simulink model "Lab_6_QRD_MVMUL"  (R2021a)
settings: Solver=VariableStepAuto  StartTime=0.0  StopTime=double(sim_length)  RelTol=1e-3
undefined symbols (not defined in the file or in its folder): AXI4, Lite
libraries: hdlBasic x118, xbsIndex_r4 x1
settings Model: Creator=ckk5  LastModifiedBy=ckk5

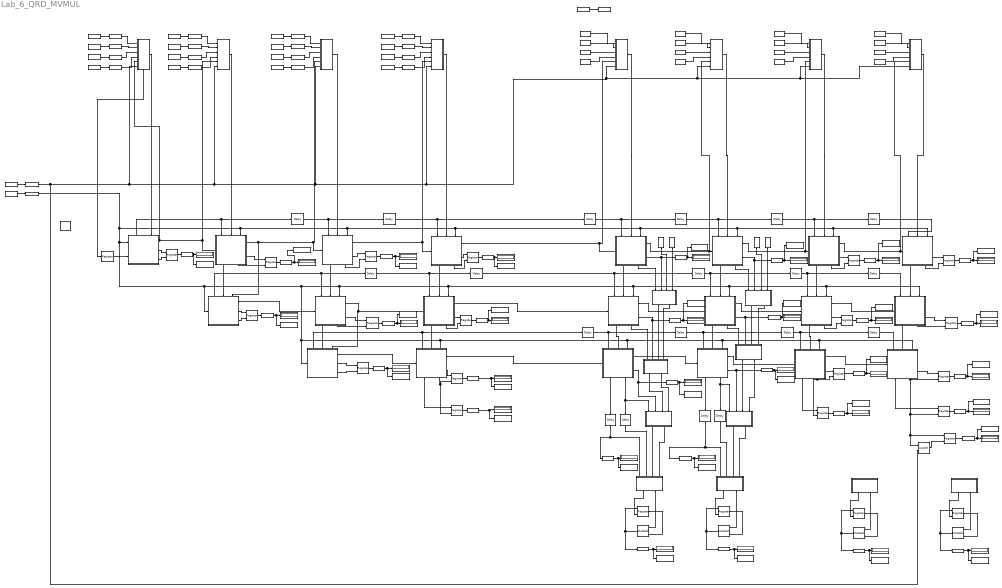
== system Lab_6_QRD_MVMUL ==
  " System Generator" : xbsIndex_r4/ System Generator  Tag=genX  xilinxfamily=zynq  part=xc7z020  speed=-1  package=clg484  synthesis_tool=Vivado  clock_wrapper=Clock Enables  directory=./netlist  proj_type=Vivado  Synth_file=Vivado Synthesis Defaults  Impl_file=Vivado Implementation Defaults  testbench=off  simulink_period=1  sysclk_period=10  dcm_input_clock_period=10  incr_netlist=off  trim_vbits=Everywhere in SubSystem  dbl_ovrd=According to Block Masks  core_generation=According to Block Masks  run_coregen=off  deprecated_control=off  eval_field=0  block_type=sysgen
  B_1 : hdlBasic/Gateway In  gui_display_data_type=Fixed-point  arith_type=Signed (2's comp)  n_bits=16  bin_pt=12  preci_type=Single  exp_width=8  frac_width=24  rows=1  columns=1  quantization="Round  (unbiased: +/- Inf)"  overflow=Saturate  period=1  UseAsADC=off  ADCChannel='1'  interface=AXI4-Lite  automatic_assignment=on  address_offset=hex2dec('00')  intf_name='array_input'  intf_description=''  default_value=0  timing_constraint=None  locs_specified=off  LOCs={}  io_standard={}  inherit_from_input=off  hdl_port=on  XmcBlockStatus=1  maskContainerNames=group4  block_type=gatewayin  block_config=sysgen:gateway_in_config  block_width_w=590  block_height_w=620  block_width=640  block_height=850
  C_{1..4} (4 alike) : hdlBasic/Gateway Out  inherit_from_input=off  hdl_port=off  rows=1  columns=1  UseAsDAC=off  DACChannel='1'  interface=AXI4-Lite  automatic_assignment=on  address_offset=hex2dec('00')  intf_name='output'  intf_description=''  timing_constraint=None  locs_specified=off  LOCs={}  io_standard={}  XmcBlockStatus=1  maskContainerNames=group4  block_type=gatewayout  block_config=sysgen:gateway_out_config  block_width_w=590  block_height_w=620  block_width=620  block_height=750
  Constant : hdlBasic/Constant  const=1.0  gui_display_data_type=Fixed-point  arith_type=Signed (2's comp)  n_bits=16  bin_pt=12  preci_type=Single  exp_width=8  frac_width=24  explicit_period=off  period=1  XmcBlockStatus=1  maskContainerNames=tabcontainer1  block_type=constant  block_config=sysgen:Constant_config
  Constant{1..4,6..9,11..14,17,19} (14 alike) : hdlBasic/Constant  const=0  gui_display_data_type=Fixed-point  arith_type=Signed (2's comp)  n_bits=16  bin_pt=12  preci_type=Single  exp_width=8  frac_width=24  explicit_period=off  period=1  XmcBlockStatus=1  maskContainerNames=tabcontainer1  block_type=constant  block_config=sysgen:Constant_config
  Constant10 : hdlBasic/Constant  const=1  gui_display_data_type=Fixed-point  arith_type=Signed (2's comp)  n_bits=16  bin_pt=12  preci_type=Single  exp_width=8  frac_width=24  explicit_period=off  period=1  XmcBlockStatus=1  maskContainerNames=tabcontainer1  block_type=constant  block_config=sysgen:Constant_config
  Constant15 : hdlBasic/Constant  const=1  gui_display_data_type=Fixed-point  arith_type=Signed (2's comp)  n_bits=16  bin_pt=12  preci_type=Single  exp_width=8  frac_width=24  explicit_period=off  period=1  XmcBlockStatus=1  maskContainerNames=tabcontainer1  block_type=constant  block_config=sysgen:Constant_config
  Constant16 : hdlBasic/Constant  const=0  gui_display_data_type=Boolean  arith_type=Boolean  n_bits=16  bin_pt=12  preci_type=Single  exp_width=8  frac_width=24  explicit_period=off  period=1  XmcBlockStatus=1  maskContainerNames=tabcontainer1  block_type=constant  block_config=sysgen:Constant_config
  Constant18 : hdlBasic/Constant  const=0  gui_display_data_type=Boolean  arith_type=Boolean  n_bits=16  bin_pt=12  preci_type=Single  exp_width=8  frac_width=24  explicit_period=off  period=1  XmcBlockStatus=1  maskContainerNames=tabcontainer1  block_type=constant  block_config=sysgen:Constant_config
  Constant5 : hdlBasic/Constant  const=1  gui_display_data_type=Fixed-point  arith_type=Signed (2's comp)  n_bits=16  bin_pt=12  preci_type=Single  exp_width=8  frac_width=24  explicit_period=off  period=1  XmcBlockStatus=1  maskContainerNames=tabcontainer1  block_type=constant  block_config=sysgen:Constant_config
  Delay{,1,4,14} (4 alike) : hdlBasic/Delay  rst=off  en=off  latency=1  reg_retiming=off  XmcBlockStatus=1  maskContainerNames=group1  block_type=delay  block_config=sysgen:Delay_config
  Delay{2..3,5..13,18..21} (15 alike) : hdlBasic/Delay  rst=off  en=off  latency=unit_L  reg_retiming=off  XmcBlockStatus=1  maskContainerNames=group1  block_type=delay  block_config=sysgen:Delay_config
  Display{,1..30} (31 alike) : Display
  From Workspace : FromWorkspace  VariableName=ap_rst  OutputAfterFinalValue=Setting to zero
  From Workspace1 : FromWorkspace  VariableName=start_new  OutputAfterFinalValue=Setting to zero
  From Workspace10 : FromWorkspace  VariableName=in_41  OutputAfterFinalValue=Setting to zero
  From Workspace11 : FromWorkspace  VariableName=in_22  OutputAfterFinalValue=Setting to zero
  From Workspace12 : FromWorkspace  VariableName=in_32  OutputAfterFinalValue=Setting to zero
  From Workspace13 : FromWorkspace  VariableName=in_33  OutputAfterFinalValue=Setting to zero
  From Workspace14 : FromWorkspace  VariableName=in_44  OutputAfterFinalValue=Setting to zero
  From Workspace15 : FromWorkspace  VariableName=in_14  OutputAfterFinalValue=Setting to zero
  From Workspace16 : FromWorkspace  VariableName=in_24  OutputAfterFinalValue=Setting to zero
  From Workspace17 : FromWorkspace  VariableName=in_34  OutputAfterFinalValue=Setting to zero
  From Workspace18 : FromWorkspace  VariableName=B_1  OutputAfterFinalValue=Setting to zero
  From Workspace2 : FromWorkspace  VariableName=in_43  OutputAfterFinalValue=Setting to zero
  From Workspace3 : FromWorkspace  VariableName=in_42  OutputAfterFinalValue=Setting to zero
  From Workspace4 : FromWorkspace  VariableName=in_13  OutputAfterFinalValue=Setting to zero
  From Workspace5 : FromWorkspace  VariableName=in_23  OutputAfterFinalValue=Setting to zero
  From Workspace6 : FromWorkspace  VariableName=in_11  OutputAfterFinalValue=Setting to zero
  From Workspace7 : FromWorkspace  VariableName=in_12  OutputAfterFinalValue=Setting to zero
  From Workspace8 : FromWorkspace  VariableName=in_21  OutputAfterFinalValue=Setting to zero
  From Workspace9 : FromWorkspace  VariableName=in_31  OutputAfterFinalValue=Setting to zero
  Logical3 : hdlBasic/Logical  logical_function=OR  inputs=2  en=off  latency=0  precision=Full  arith_type=Unsigned  n_bits=16  bin_pt=0  align_bp=on  overflow=[]  quantization=[]  XmcBlockStatus=1  maskContainerNames=tabcontainer1  block_type=logical  block_config=sysgen:Logical_config
  MultAdd{,1..3} (4 alike) : hdlBasic/MultAdd  mode=Addition  en=off  latency=0  precision=Full  arith_type=Unsigned  n_bits=16  bin_pt=14  XmcBlockStatus=1  maskContainerNames=tabcontainer1  block_type=multadd  block_config=sysgen:MultAdd_config
  Q_1 : hdlBasic/Gateway Out  inherit_from_input=off  hdl_port=on  rows=1  columns=1  UseAsDAC=off  DACChannel='1'  interface=AXI4-Lite  automatic_assignment=on  address_offset=hex2dec('00')  intf_name='control'  intf_description=''  timing_constraint=None  locs_specified=off  LOCs={}  io_standard={}  XmcBlockStatus=1  maskContainerNames=group4  block_type=gatewayout  block_config=sysgen:gateway_out_config  block_width_w=590  block_height_w=620  block_width=620  block_height=750
  Q_{11,21..22,31..32,41} (6 alike) : hdlBasic/Gateway Out  inherit_from_input=off  hdl_port=off  rows=1  columns=1  UseAsDAC=off  DACChannel='1'  interface=None  automatic_assignment=on  address_offset=hex2dec('00')  intf_name='output'  intf_description=''  timing_constraint=None  locs_specified=off  LOCs={}  io_standard={}  XmcBlockStatus=1  maskContainerNames=group4  block_type=gatewayout  block_config=sysgen:gateway_out_config  block_width_w=590  block_height_w=620  block_width=620  block_height=750
  Q_{12..14,23..24,33..34,43..44} (9 alike) : hdlBasic/Gateway Out  inherit_from_input=off  hdl_port=on  rows=1  columns=1  UseAsDAC=off  DACChannel='1'  interface=AXI4-Lite  automatic_assignment=on  address_offset=hex2dec('00')  intf_name='output'  intf_description=''  timing_constraint=None  locs_specified=off  LOCs={}  io_standard={}  XmcBlockStatus=1  maskContainerNames=group4  block_type=gatewayout  block_config=sysgen:gateway_out_config  block_width_w=590  block_height_w=620  block_width=620  block_height=750
  Q_42 : hdlBasic/Gateway Out  inherit_from_input=off  hdl_port=off  rows=1  columns=1  UseAsDAC=off  DACChannel='1'  interface=None  automatic_assignment=off  address_offset=hex2dec('00')  intf_name='output'  intf_description=''  timing_constraint=None  locs_specified=off  LOCs={}  io_standard={}  XmcBlockStatus=1  maskContainerNames=group4  block_type=gatewayout  block_config=sysgen:gateway_out_config  block_width_w=590  block_height_w=620  block_width=620  block_height=750
  R_{11..14,22..24,33..34,44} (10 alike) : hdlBasic/Gateway Out  inherit_from_input=off  hdl_port=on  rows=1  columns=1  UseAsDAC=off  DACChannel='1'  interface=AXI4-Lite  automatic_assignment=on  address_offset=hex2dec('00')  intf_name='output'  intf_description=''  timing_constraint=None  locs_specified=off  LOCs={}  io_standard={}  XmcBlockStatus=1  maskContainerNames=group4  block_type=gatewayout  block_config=sysgen:gateway_out_config  block_width_w=590  block_height_w=620  block_width=620  block_height=750
  Register{,1..4,6..14,16..18,20..21,24..25,27..28} (23 alike) : hdlBasic/Register  init=0  rst=off  en=on  XmcBlockStatus=1  maskContainerNames=tabcontainer1  block_type=register  block_config=sysgen:Register_config
  Register26 : hdlBasic/Register  init=0  rst=off  en=off  XmcBlockStatus=1  maskContainerNames=tabcontainer1  block_type=register  block_config=sysgen:Register_config
  Subsystem{,1..7} (8 alike) : Subsystem  ReferencedSubsystem=input_muxer
      Subsystem settings: PortSchema="{\"entries\":[{\"content\":{\"sides\":[{\"content\":{\"connectorIds\":[\"In1\",\"In2\",\"In3\",\"In4\",\"In5\",\"In6\"]},\"type\":\"ConnectorPlacement.EquallySpacedRectSide\",\"uuid\":\"c9659870-197e-4708-9e56-aa8d60ec2132\"},{\"content\":{\"connectorIds\":[\"Out1\"],\"side\":\"RIGHT\"},\"type\":\"ConnectorPlacement.EquallySpacedRectSide\",\"uuid\":\"f9d7c189-098f-4a24-828d-c7ef82e0ce16\"},{\"content\":{\"connectorIds\":[],\"side\":\"TOP\"},\"type\":\"ConnectorPlacement.EquallySpacedRectSide\",\"uuid\":\"5053940a-c387-4687-a81e-c4b094664b8d\"},{\"content\":{\"connectorIds\":[\"Out2\"],\"side\":\"BOTTOM\"},\"type\":\"ConnectorPlacement.EquallySpacedRectSide\",\"uuid\":\"4f75bbb3-aea6-4cac-bddf-f1fd262beda3\"}]},\"type\":\"ConnectorPlacement.EquallySpacedConnector\",\"uuid\":\"5b5beda6-ba80-4093-9766-00cb89766bfd\"}],\"packageUris\":[\"http://schema.mathworks.com/mf0/Connector/R2020b\"],\"version\":\"1.0\"}"
      Subsystem1 settings: PortSchema="{\"entries\":[{\"content\":{\"sides\":[{\"content\":{\"connectorIds\":[\"In1\",\"In2\",\"In3\",\"In4\",\"In5\",\"In6\"]},\"type\":\"ConnectorPlacement.EquallySpacedRectSide\",\"uuid\":\"c9659870-197e-4708-9e56-aa8d60ec2132\"},{\"content\":{\"connectorIds\":[\"Out1\"],\"side\":\"RIGHT\"},\"type\":\"ConnectorPlacement.EquallySpacedRectSide\",\"uuid\":\"f9d7c189-098f-4a24-828d-c7ef82e0ce16\"},{\"content\":{\"connectorIds\":[],\"side\":\"TOP\"},\"type\":\"ConnectorPlacement.EquallySpacedRectSide\",\"uuid\":\"5053940a-c387-4687-a81e-c4b094664b8d\"},{\"content\":{\"connectorIds\":[\"Out2\"],\"side\":\"BOTTOM\"},\"type\":\"ConnectorPlacement.EquallySpacedRectSide\",\"uuid\":\"0386b525-0d84-489d-b1ba-c0f65ef89545\"}]},\"type\":\"ConnectorPlacement.EquallySpacedConnector\",\"uuid\":\"5b5beda6-ba80-4093-9766-00cb89766bfd\"}],\"packageUris\":[\"http://schema.mathworks.com/mf0/Connector/R2020b\"],\"version\":\"1.0\"}"
      Subsystem2 settings: PortSchema="{\"entries\":[{\"content\":{\"sides\":[{\"content\":{\"connectorIds\":[\"In1\",\"In2\",\"In3\",\"In4\",\"In5\",\"In6\"]},\"type\":\"ConnectorPlacement.EquallySpacedRectSide\",\"uuid\":\"c9659870-197e-4708-9e56-aa8d60ec2132\"},{\"content\":{\"connectorIds\":[\"Out1\"],\"side\":\"RIGHT\"},\"type\":\"ConnectorPlacement.EquallySpacedRectSide\",\"uuid\":\"f9d7c189-098f-4a24-828d-c7ef82e0ce16\"},{\"content\":{\"connectorIds\":[],\"side\":\"TOP\"},\"type\":\"ConnectorPlacement.EquallySpacedRectSide\",\"uuid\":\"5053940a-c387-4687-a81e-c4b094664b8d\"},{\"content\":{\"connectorIds\":[\"Out2\"],\"side\":\"BOTTOM\"},\"type\":\"ConnectorPlacement.EquallySpacedRectSide\",\"uuid\":\"0b7a346d-dc43-4519-a9aa-7889b337343a\"}]},\"type\":\"ConnectorPlacement.EquallySpacedConnector\",\"uuid\":\"5b5beda6-ba80-4093-9766-00cb89766bfd\"}],\"packageUris\":[\"http://schema.mathworks.com/mf0/Connector/R2020b\"],\"version\":\"1.0\"}"
      Subsystem3 settings: PortSchema="{\"entries\":[{\"content\":{\"sides\":[{\"content\":{\"connectorIds\":[\"In1\",\"In2\",\"In3\",\"In4\",\"In5\",\"In6\"]},\"type\":\"ConnectorPlacement.EquallySpacedRectSide\",\"uuid\":\"c9659870-197e-4708-9e56-aa8d60ec2132\"},{\"content\":{\"connectorIds\":[\"Out1\"],\"side\":\"RIGHT\"},\"type\":\"ConnectorPlacement.EquallySpacedRectSide\",\"uuid\":\"f9d7c189-098f-4a24-828d-c7ef82e0ce16\"},{\"content\":{\"connectorIds\":[],\"side\":\"TOP\"},\"type\":\"ConnectorPlacement.EquallySpacedRectSide\",\"uuid\":\"5053940a-c387-4687-a81e-c4b094664b8d\"},{\"content\":{\"connectorIds\":[\"Out2\"],\"side\":\"BOTTOM\"},\"type\":\"ConnectorPlacement.EquallySpacedRectSide\",\"uuid\":\"96ca4152-851a-4b7b-aabe-a144e8b0fd46\"}]},\"type\":\"ConnectorPlacement.EquallySpacedConnector\",\"uuid\":\"5b5beda6-ba80-4093-9766-00cb89766bfd\"}],\"packageUris\":[\"http://schema.mathworks.com/mf0/Connector/R2020b\"],\"version\":\"1.0\"}"
      Subsystem4 settings: PortSchema="{\"entries\":[{\"content\":{\"sides\":[{\"content\":{\"connectorIds\":[\"In1\",\"In2\",\"In3\",\"In4\",\"In5\",\"In6\"]},\"type\":\"ConnectorPlacement.EquallySpacedRectSide\",\"uuid\":\"c9659870-197e-4708-9e56-aa8d60ec2132\"},{\"content\":{\"connectorIds\":[\"Out1\"],\"side\":\"RIGHT\"},\"type\":\"ConnectorPlacement.EquallySpacedRectSide\",\"uuid\":\"f9d7c189-098f-4a24-828d-c7ef82e0ce16\"},{\"content\":{\"connectorIds\":[],\"side\":\"TOP\"},\"type\":\"ConnectorPlacement.EquallySpacedRectSide\",\"uuid\":\"5053940a-c387-4687-a81e-c4b094664b8d\"},{\"content\":{\"connectorIds\":[\"Out2\"],\"side\":\"BOTTOM\"},\"type\":\"ConnectorPlacement.EquallySpacedRectSide\",\"uuid\":\"96ca4152-851a-4b7b-aabe-a144e8b0fd46\"}]},\"type\":\"ConnectorPlacement.EquallySpacedConnector\",\"uuid\":\"5b5beda6-ba80-4093-9766-00cb89766bfd\"}],\"packageUris\":[\"http://schema.mathworks.com/mf0/Connector/R2020b\"],\"version\":\"1.0\"}"
      Subsystem5 settings: PortSchema="{\"entries\":[{\"content\":{\"sides\":[{\"content\":{\"connectorIds\":[\"In1\",\"In2\",\"In3\",\"In4\",\"In5\",\"In6\"]},\"type\":\"ConnectorPlacement.EquallySpacedRectSide\",\"uuid\":\"c9659870-197e-4708-9e56-aa8d60ec2132\"},{\"content\":{\"connectorIds\":[\"Out1\"],\"side\":\"RIGHT\"},\"type\":\"ConnectorPlacement.EquallySpacedRectSide\",\"uuid\":\"f9d7c189-098f-4a24-828d-c7ef82e0ce16\"},{\"content\":{\"connectorIds\":[],\"side\":\"TOP\"},\"type\":\"ConnectorPlacement.EquallySpacedRectSide\",\"uuid\":\"5053940a-c387-4687-a81e-c4b094664b8d\"},{\"content\":{\"connectorIds\":[\"Out2\"],\"side\":\"BOTTOM\"},\"type\":\"ConnectorPlacement.EquallySpacedRectSide\",\"uuid\":\"96ca4152-851a-4b7b-aabe-a144e8b0fd46\"}]},\"type\":\"ConnectorPlacement.EquallySpacedConnector\",\"uuid\":\"5b5beda6-ba80-4093-9766-00cb89766bfd\"}],\"packageUris\":[\"http://schema.mathworks.com/mf0/Connector/R2020b\"],\"version\":\"1.0\"}"
      Subsystem6 settings: PortSchema="{\"entries\":[{\"content\":{\"sides\":[{\"content\":{\"connectorIds\":[\"In1\",\"In2\",\"In3\",\"In4\",\"In5\",\"In6\"]},\"type\":\"ConnectorPlacement.EquallySpacedRectSide\",\"uuid\":\"c9659870-197e-4708-9e56-aa8d60ec2132\"},{\"content\":{\"connectorIds\":[\"Out1\"],\"side\":\"RIGHT\"},\"type\":\"ConnectorPlacement.EquallySpacedRectSide\",\"uuid\":\"f9d7c189-098f-4a24-828d-c7ef82e0ce16\"},{\"content\":{\"connectorIds\":[],\"side\":\"TOP\"},\"type\":\"ConnectorPlacement.EquallySpacedRectSide\",\"uuid\":\"5053940a-c387-4687-a81e-c4b094664b8d\"},{\"content\":{\"connectorIds\":[\"Out2\"],\"side\":\"BOTTOM\"},\"type\":\"ConnectorPlacement.EquallySpacedRectSide\",\"uuid\":\"96ca4152-851a-4b7b-aabe-a144e8b0fd46\"}]},\"type\":\"ConnectorPlacement.EquallySpacedConnector\",\"uuid\":\"5b5beda6-ba80-4093-9766-00cb89766bfd\"}],\"packageUris\":[\"http://schema.mathworks.com/mf0/Connector/R2020b\"],\"version\":\"1.0\"}"
      Subsystem7 settings: PortSchema="{\"entries\":[{\"content\":{\"sides\":[{\"content\":{\"connectorIds\":[\"In1\",\"In2\",\"In3\",\"In4\",\"In5\",\"In6\"]},\"type\":\"ConnectorPlacement.EquallySpacedRectSide\",\"uuid\":\"c9659870-197e-4708-9e56-aa8d60ec2132\"},{\"content\":{\"connectorIds\":[\"Out1\"],\"side\":\"RIGHT\"},\"type\":\"ConnectorPlacement.EquallySpacedRectSide\",\"uuid\":\"f9d7c189-098f-4a24-828d-c7ef82e0ce16\"},{\"content\":{\"connectorIds\":[],\"side\":\"TOP\"},\"type\":\"ConnectorPlacement.EquallySpacedRectSide\",\"uuid\":\"5053940a-c387-4687-a81e-c4b094664b8d\"},{\"content\":{\"connectorIds\":[\"Out2\"],\"side\":\"BOTTOM\"},\"type\":\"ConnectorPlacement.EquallySpacedRectSide\",\"uuid\":\"96ca4152-851a-4b7b-aabe-a144e8b0fd46\"}]},\"type\":\"ConnectorPlacement.EquallySpacedConnector\",\"uuid\":\"5b5beda6-ba80-4093-9766-00cb89766bfd\"}],\"packageUris\":[\"http://schema.mathworks.com/mf0/Connector/R2020b\"],\"version\":\"1.0\"}"
  Subsystem Reference : Subsystem  ReferencedSubsystem=ATAN_static
      settings: PortSchema="{\"entries\":[{\"content\":{\"sides\":[{\"content\":{\"connectorIds\":[\"In1\"]},\"type\":\"ConnectorPlacement.EquallySpacedRectSide\",\"uuid\":\"e73d0d7d-03bc-4d00-801b-b8c760b16be4\"},{\"content\":{\"connectorIds\":[\"Out1\",\"Out3\",\"Out4\"],\"side\":\"RIGHT\"},\"type\":\"ConnectorPlacement.EquallySpacedRectSide\",\"uuid\":\"fb412951-8b1f-47f8-8fed-40e91e78b205\"},{\"content\":{\"connectorIds\":[\"Out2\",\"In3\",\"In2\"],\"side\":\"TOP\"},\"type\":\"ConnectorPlacement.EquallySpacedRectSide\",\"uuid\":\"8225374e-1161-490d-99ec-3bdc7c7ef343\"},{\"content\":{\"connectorIds\":[\"Out5\"],\"side\":\"BOTTOM\"},\"type\":\"ConnectorPlacement.EquallySpacedRectSide\",\"uuid\":\"cef28eec-a681-4ab7-b320-ffc64443d109\"}]},\"type\":\"ConnectorPlacement.EquallySpacedConnector\",\"uuid\":\"16b5b7a4-aca7-4d8e-a872-8aaff24fa59b\"}],\"packageUris\":[\"http://schema.mathworks.com/mf0/Connector/R2020b\"],\"version\":\"1.0\"}"
  Subsystem Reference1 : Subsystem  ReferencedSubsystem=ATAN_static
      settings: PortSchema="{\"entries\":[{\"content\":{\"sides\":[{\"content\":{\"connectorIds\":[\"In1\",\"In2\"]},\"type\":\"ConnectorPlacement.EquallySpacedRectSide\",\"uuid\":\"e73d0d7d-03bc-4d00-801b-b8c760b16be4\"},{\"content\":{\"connectorIds\":[\"Out1\",\"Out3\",\"Out4\"],\"side\":\"RIGHT\"},\"type\":\"ConnectorPlacement.EquallySpacedRectSide\",\"uuid\":\"fb412951-8b1f-47f8-8fed-40e91e78b205\"},{\"content\":{\"connectorIds\":[\"Out2\",\"In3\"],\"side\":\"TOP\"},\"type\":\"ConnectorPlacement.EquallySpacedRectSide\",\"uuid\":\"8225374e-1161-490d-99ec-3bdc7c7ef343\"},{\"content\":{\"connectorIds\":[\"Out5\"],\"side\":\"BOTTOM\"},\"type\":\"ConnectorPlacement.EquallySpacedRectSide\",\"uuid\":\"cef28eec-a681-4ab7-b320-ffc64443d109\"}]},\"type\":\"ConnectorPlacement.EquallySpacedConnector\",\"uuid\":\"16b5b7a4-aca7-4d8e-a872-8aaff24fa59b\"}],\"packageUris\":[\"http://schema.mathworks.com/mf0/Connector/R2020b\"],\"version\":\"1.0\"}"
  Subsystem Reference{2,4..20} (18 alike) : Subsystem  ReferencedSubsystem=ROT_static
      settings: PortSchema="{\"entries\":[{\"content\":{\"sides\":[{\"content\":{\"connectorIds\":[\"In2\"]},\"type\":\"ConnectorPlacement.EquallySpacedRectSide\",\"uuid\":\"e73d0d7d-03bc-4d00-801b-b8c760b16be4\"},{\"content\":{\"connectorIds\":[\"Out1\",\"Out3\"],\"side\":\"RIGHT\"},\"type\":\"ConnectorPlacement.EquallySpacedRectSide\",\"uuid\":\"fb412951-8b1f-47f8-8fed-40e91e78b205\"},{\"content\":{\"connectorIds\":[\"In3\",\"In4\",\"In1\"],\"side\":\"TOP\"},\"type\":\"ConnectorPlacement.EquallySpacedRectSide\",\"uuid\":\"8225374e-1161-490d-99ec-3bdc7c7ef343\"},{\"content\":{\"connectorIds\":[\"Out2\",\"Out4\"],\"side\":\"BOTTOM\"},\"type\":\"ConnectorPlacement.EquallySpacedRectSide\",\"uuid\":\"cef28eec-a681-4ab7-b320-ffc64443d109\"}]},\"type\":\"ConnectorPlacement.EquallySpacedConnector\",\"uuid\":\"16b5b7a4-aca7-4d8e-a872-8aaff24fa59b\"}],\"packageUris\":[\"http://schema.mathworks.com/mf0/Connector/R2020b\"],\"version\":\"1.0\"}"
  Subsystem Reference3 : Subsystem  ReferencedSubsystem=ATAN_static
      settings: PortSchema="{\"entries\":[{\"content\":{\"sides\":[{\"content\":{\"connectorIds\":[\"In1\"]},\"type\":\"ConnectorPlacement.EquallySpacedRectSide\",\"uuid\":\"e73d0d7d-03bc-4d00-801b-b8c760b16be4\"},{\"content\":{\"connectorIds\":[\"Out1\",\"Out3\",\"Out4\"],\"side\":\"RIGHT\"},\"type\":\"ConnectorPlacement.EquallySpacedRectSide\",\"uuid\":\"fb412951-8b1f-47f8-8fed-40e91e78b205\"},{\"content\":{\"connectorIds\":[\"Out2\",\"In3\",\"In2\"],\"side\":\"TOP\"},\"type\":\"ConnectorPlacement.EquallySpacedRectSide\",\"uuid\":\"8225374e-1161-490d-99ec-3bdc7c7ef343\"},{\"content\":{\"connectorIds\":[\"Out5\"],\"side\":\"BOTTOM\"},\"type\":\"ConnectorPlacement.EquallySpacedRectSide\",\"uuid\":\"cef28eec-a681-4ab7-b320-ffc64443d109\"}]},\"type\":\"ConnectorPlacement.EquallySpacedConnector\",\"uuid\":\"16b5b7a4-aca7-4d8e-a872-8aaff24fa59b\"}],\"packageUris\":[\"http://schema.mathworks.com/mf0/Connector/R2020b\"],\"version\":\"1.0\"}"
  Subsystem{8..17} (10 alike) : Subsystem  ReferencedSubsystem=Output_Selector_Simple
      Subsystem10 settings: PortSchema="{\"entries\":[{\"content\":{\"sides\":[{\"content\":{\"connectorIds\":[]},\"type\":\"ConnectorPlacement.EquallySpacedRectSide\",\"uuid\":\"f96c7e86-64a4-4252-abea-b711e367158a\"},{\"content\":{\"connectorIds\":[],\"side\":\"RIGHT\"},\"type\":\"ConnectorPlacement.EquallySpacedRectSide\",\"uuid\":\"0939b534-8e75-43bd-89b2-3b8c6cf8d932\"},{\"content\":{\"connectorIds\":[\"In2\",\"In1\",\"In4\",\"In3\"],\"side\":\"TOP\"},\"type\":\"ConnectorPlacement.EquallySpacedRectSide\",\"uuid\":\"1f2daeb6-2bdf-409b-a45b-4c9e00127dcc\"},{\"content\":{\"connectorIds\":[\"Out2\",\"Out1\"],\"side\":\"BOTTOM\"},\"type\":\"ConnectorPlacement.EquallySpacedRectSide\",\"uuid\":\"39a7ca2e-4955-4af4-a4e8-230b89e841c3\"}]},\"type\":\"ConnectorPlacement.EquallySpacedConnector\",\"uuid\":\"4fbf931e-4755-4fcf-8161-08b087bf3058\"}],\"packageUris\":[\"http://schema.mathworks.com/mf0/Connector/R2020b\"],\"version\":\"1.0\"}"
      Subsystem11 settings: PortSchema="{\"entries\":[{\"content\":{\"sides\":[{\"content\":{\"connectorIds\":[]},\"type\":\"ConnectorPlacement.EquallySpacedRectSide\",\"uuid\":\"f96c7e86-64a4-4252-abea-b711e367158a\"},{\"content\":{\"connectorIds\":[],\"side\":\"RIGHT\"},\"type\":\"ConnectorPlacement.EquallySpacedRectSide\",\"uuid\":\"0939b534-8e75-43bd-89b2-3b8c6cf8d932\"},{\"content\":{\"connectorIds\":[\"In2\",\"In1\",\"In4\",\"In3\"],\"side\":\"TOP\"},\"type\":\"ConnectorPlacement.EquallySpacedRectSide\",\"uuid\":\"1f2daeb6-2bdf-409b-a45b-4c9e00127dcc\"},{\"content\":{\"connectorIds\":[\"Out2\",\"Out1\"],\"side\":\"BOTTOM\"},\"type\":\"ConnectorPlacement.EquallySpacedRectSide\",\"uuid\":\"39a7ca2e-4955-4af4-a4e8-230b89e841c3\"}]},\"type\":\"ConnectorPlacement.EquallySpacedConnector\",\"uuid\":\"4fbf931e-4755-4fcf-8161-08b087bf3058\"}],\"packageUris\":[\"http://schema.mathworks.com/mf0/Connector/R2020b\"],\"version\":\"1.0\"}"
      Subsystem12 settings: PortSchema="{\"entries\":[{\"content\":{\"sides\":[{\"content\":{\"connectorIds\":[]},\"type\":\"ConnectorPlacement.EquallySpacedRectSide\",\"uuid\":\"f96c7e86-64a4-4252-abea-b711e367158a\"},{\"content\":{\"connectorIds\":[],\"side\":\"RIGHT\"},\"type\":\"ConnectorPlacement.EquallySpacedRectSide\",\"uuid\":\"0939b534-8e75-43bd-89b2-3b8c6cf8d932\"},{\"content\":{\"connectorIds\":[\"In1\",\"In2\",\"In4\",\"In3\"],\"side\":\"TOP\"},\"type\":\"ConnectorPlacement.EquallySpacedRectSide\",\"uuid\":\"1f2daeb6-2bdf-409b-a45b-4c9e00127dcc\"},{\"content\":{\"connectorIds\":[\"Out2\",\"Out1\"],\"side\":\"BOTTOM\"},\"type\":\"ConnectorPlacement.EquallySpacedRectSide\",\"uuid\":\"39a7ca2e-4955-4af4-a4e8-230b89e841c3\"}]},\"type\":\"ConnectorPlacement.EquallySpacedConnector\",\"uuid\":\"4fbf931e-4755-4fcf-8161-08b087bf3058\"}],\"packageUris\":[\"http://schema.mathworks.com/mf0/Connector/R2020b\"],\"version\":\"1.0\"}"
      Subsystem13 settings: PortSchema="{\"entries\":[{\"content\":{\"sides\":[{\"content\":{\"connectorIds\":[]},\"type\":\"ConnectorPlacement.EquallySpacedRectSide\",\"uuid\":\"f96c7e86-64a4-4252-abea-b711e367158a\"},{\"content\":{\"connectorIds\":[],\"side\":\"RIGHT\"},\"type\":\"ConnectorPlacement.EquallySpacedRectSide\",\"uuid\":\"0939b534-8e75-43bd-89b2-3b8c6cf8d932\"},{\"content\":{\"connectorIds\":[\"In1\",\"In2\",\"In4\",\"In3\"],\"side\":\"TOP\"},\"type\":\"ConnectorPlacement.EquallySpacedRectSide\",\"uuid\":\"1f2daeb6-2bdf-409b-a45b-4c9e00127dcc\"},{\"content\":{\"connectorIds\":[\"Out2\",\"Out1\"],\"side\":\"BOTTOM\"},\"type\":\"ConnectorPlacement.EquallySpacedRectSide\",\"uuid\":\"39a7ca2e-4955-4af4-a4e8-230b89e841c3\"}]},\"type\":\"ConnectorPlacement.EquallySpacedConnector\",\"uuid\":\"4fbf931e-4755-4fcf-8161-08b087bf3058\"}],\"packageUris\":[\"http://schema.mathworks.com/mf0/Connector/R2020b\"],\"version\":\"1.0\"}"
      Subsystem14 settings: PortSchema="{\"entries\":[{\"content\":{\"sides\":[{\"content\":{\"connectorIds\":[]},\"type\":\"ConnectorPlacement.EquallySpacedRectSide\",\"uuid\":\"f96c7e86-64a4-4252-abea-b711e367158a\"},{\"content\":{\"connectorIds\":[],\"side\":\"RIGHT\"},\"type\":\"ConnectorPlacement.EquallySpacedRectSide\",\"uuid\":\"0939b534-8e75-43bd-89b2-3b8c6cf8d932\"},{\"content\":{\"connectorIds\":[\"In1\",\"In2\",\"In4\",\"In3\"],\"side\":\"TOP\"},\"type\":\"ConnectorPlacement.EquallySpacedRectSide\",\"uuid\":\"1f2daeb6-2bdf-409b-a45b-4c9e00127dcc\"},{\"content\":{\"connectorIds\":[\"Out2\",\"Out1\"],\"side\":\"BOTTOM\"},\"type\":\"ConnectorPlacement.EquallySpacedRectSide\",\"uuid\":\"39a7ca2e-4955-4af4-a4e8-230b89e841c3\"}]},\"type\":\"ConnectorPlacement.EquallySpacedConnector\",\"uuid\":\"4fbf931e-4755-4fcf-8161-08b087bf3058\"}],\"packageUris\":[\"http://schema.mathworks.com/mf0/Connector/R2020b\"],\"version\":\"1.0\"}"
      Subsystem15 settings: PortSchema="{\"entries\":[{\"content\":{\"sides\":[{\"content\":{\"connectorIds\":[]},\"type\":\"ConnectorPlacement.EquallySpacedRectSide\",\"uuid\":\"f96c7e86-64a4-4252-abea-b711e367158a\"},{\"content\":{\"connectorIds\":[],\"side\":\"RIGHT\"},\"type\":\"ConnectorPlacement.EquallySpacedRectSide\",\"uuid\":\"0939b534-8e75-43bd-89b2-3b8c6cf8d932\"},{\"content\":{\"connectorIds\":[\"In2\",\"In1\",\"In4\",\"In3\"],\"side\":\"TOP\"},\"type\":\"ConnectorPlacement.EquallySpacedRectSide\",\"uuid\":\"1f2daeb6-2bdf-409b-a45b-4c9e00127dcc\"},{\"content\":{\"connectorIds\":[\"Out2\",\"Out1\"],\"side\":\"BOTTOM\"},\"type\":\"ConnectorPlacement.EquallySpacedRectSide\",\"uuid\":\"39a7ca2e-4955-4af4-a4e8-230b89e841c3\"}]},\"type\":\"ConnectorPlacement.EquallySpacedConnector\",\"uuid\":\"4fbf931e-4755-4fcf-8161-08b087bf3058\"}],\"packageUris\":[\"http://schema.mathworks.com/mf0/Connector/R2020b\"],\"version\":\"1.0\"}"
      Subsystem16 settings: PortSchema="{\"entries\":[{\"content\":{\"sides\":[{\"content\":{\"connectorIds\":[]},\"type\":\"ConnectorPlacement.EquallySpacedRectSide\",\"uuid\":\"f96c7e86-64a4-4252-abea-b711e367158a\"},{\"content\":{\"connectorIds\":[],\"side\":\"RIGHT\"},\"type\":\"ConnectorPlacement.EquallySpacedRectSide\",\"uuid\":\"0939b534-8e75-43bd-89b2-3b8c6cf8d932\"},{\"content\":{\"connectorIds\":[\"In2\",\"In1\",\"In4\",\"In3\"],\"side\":\"TOP\"},\"type\":\"ConnectorPlacement.EquallySpacedRectSide\",\"uuid\":\"1f2daeb6-2bdf-409b-a45b-4c9e00127dcc\"},{\"content\":{\"connectorIds\":[\"Out2\",\"Out1\"],\"side\":\"BOTTOM\"},\"type\":\"ConnectorPlacement.EquallySpacedRectSide\",\"uuid\":\"39a7ca2e-4955-4af4-a4e8-230b89e841c3\"}]},\"type\":\"ConnectorPlacement.EquallySpacedConnector\",\"uuid\":\"4fbf931e-4755-4fcf-8161-08b087bf3058\"}],\"packageUris\":[\"http://schema.mathworks.com/mf0/Connector/R2020b\"],\"version\":\"1.0\"}"
      Subsystem17 settings: PortSchema="{\"entries\":[{\"content\":{\"sides\":[{\"content\":{\"connectorIds\":[]},\"type\":\"ConnectorPlacement.EquallySpacedRectSide\",\"uuid\":\"f96c7e86-64a4-4252-abea-b711e367158a\"},{\"content\":{\"connectorIds\":[],\"side\":\"RIGHT\"},\"type\":\"ConnectorPlacement.EquallySpacedRectSide\",\"uuid\":\"0939b534-8e75-43bd-89b2-3b8c6cf8d932\"},{\"content\":{\"connectorIds\":[\"In2\",\"In1\",\"In4\",\"In3\"],\"side\":\"TOP\"},\"type\":\"ConnectorPlacement.EquallySpacedRectSide\",\"uuid\":\"1f2daeb6-2bdf-409b-a45b-4c9e00127dcc\"},{\"content\":{\"connectorIds\":[\"Out2\",\"Out1\"],\"side\":\"BOTTOM\"},\"type\":\"ConnectorPlacement.EquallySpacedRectSide\",\"uuid\":\"39a7ca2e-4955-4af4-a4e8-230b89e841c3\"}]},\"type\":\"ConnectorPlacement.EquallySpacedConnector\",\"uuid\":\"4fbf931e-4755-4fcf-8161-08b087bf3058\"}],\"packageUris\":[\"http://schema.mathworks.com/mf0/Connector/R2020b\"],\"version\":\"1.0\"}"
      Subsystem8 settings: PortSchema="{\"entries\":[{\"content\":{\"sides\":[{\"content\":{\"connectorIds\":[]},\"type\":\"ConnectorPlacement.EquallySpacedRectSide\",\"uuid\":\"f96c7e86-64a4-4252-abea-b711e367158a\"},{\"content\":{\"connectorIds\":[],\"side\":\"RIGHT\"},\"type\":\"ConnectorPlacement.EquallySpacedRectSide\",\"uuid\":\"0939b534-8e75-43bd-89b2-3b8c6cf8d932\"},{\"content\":{\"connectorIds\":[\"In1\",\"In2\",\"In4\",\"In3\"],\"side\":\"TOP\"},\"type\":\"ConnectorPlacement.EquallySpacedRectSide\",\"uuid\":\"1f2daeb6-2bdf-409b-a45b-4c9e00127dcc\"},{\"content\":{\"connectorIds\":[\"Out2\",\"Out1\"],\"side\":\"BOTTOM\"},\"type\":\"ConnectorPlacement.EquallySpacedRectSide\",\"uuid\":\"39a7ca2e-4955-4af4-a4e8-230b89e841c3\"}]},\"type\":\"ConnectorPlacement.EquallySpacedConnector\",\"uuid\":\"4fbf931e-4755-4fcf-8161-08b087bf3058\"}],\"packageUris\":[\"http://schema.mathworks.com/mf0/Connector/R2020b\"],\"version\":\"1.0\"}"
      Subsystem9 settings: PortSchema="{\"entries\":[{\"content\":{\"sides\":[{\"content\":{\"connectorIds\":[]},\"type\":\"ConnectorPlacement.EquallySpacedRectSide\",\"uuid\":\"f96c7e86-64a4-4252-abea-b711e367158a\"},{\"content\":{\"connectorIds\":[],\"side\":\"RIGHT\"},\"type\":\"ConnectorPlacement.EquallySpacedRectSide\",\"uuid\":\"0939b534-8e75-43bd-89b2-3b8c6cf8d932\"},{\"content\":{\"connectorIds\":[\"In2\",\"In1\",\"In4\",\"In3\"],\"side\":\"TOP\"},\"type\":\"ConnectorPlacement.EquallySpacedRectSide\",\"uuid\":\"1f2daeb6-2bdf-409b-a45b-4c9e00127dcc\"},{\"content\":{\"connectorIds\":[\"Out2\",\"Out1\"],\"side\":\"BOTTOM\"},\"type\":\"ConnectorPlacement.EquallySpacedRectSide\",\"uuid\":\"39a7ca2e-4955-4af4-a4e8-230b89e841c3\"}]},\"type\":\"ConnectorPlacement.EquallySpacedConnector\",\"uuid\":\"4fbf931e-4755-4fcf-8161-08b087bf3058\"}],\"packageUris\":[\"http://schema.mathworks.com/mf0/Connector/R2020b\"],\"version\":\"1.0\"}"
  To Workspace : ToWorkspace  VariableName=R_11  SaveFormat=Timeseries  SampleTime=-1
  To Workspace1 : ToWorkspace  VariableName=R_12  SaveFormat=Timeseries  SampleTime=-1
  To Workspace10 : ToWorkspace  VariableName=Q_11  SaveFormat=Timeseries  SampleTime=-1
  To Workspace11 : ToWorkspace  VariableName=Q_21  SaveFormat=Timeseries  SampleTime=-1
  To Workspace12 : ToWorkspace  VariableName=Q_31  SaveFormat=Timeseries  SampleTime=-1
  To Workspace13 : ToWorkspace  VariableName=Q_41  SaveFormat=Timeseries  SampleTime=-1
  To Workspace14 : ToWorkspace  VariableName=Q_42  SaveFormat=Timeseries  SampleTime=-1
  To Workspace15 : ToWorkspace  VariableName=Q_32  SaveFormat=Timeseries  SampleTime=-1
  To Workspace16 : ToWorkspace  VariableName=Q_22  SaveFormat=Timeseries  SampleTime=-1
  To Workspace17 : ToWorkspace  VariableName=Q_12  SaveFormat=Timeseries  SampleTime=-1
  To Workspace18 : ToWorkspace  VariableName=Q_13  SaveFormat=Timeseries  SampleTime=-1
  To Workspace19 : ToWorkspace  VariableName=Q_23  SaveFormat=Timeseries  SampleTime=-1
  To Workspace2 : ToWorkspace  VariableName=R_22  SaveFormat=Timeseries  SampleTime=-1
  To Workspace20 : ToWorkspace  VariableName=Q_33  SaveFormat=Timeseries  SampleTime=-1
  To Workspace21 : ToWorkspace  VariableName=Q_43  SaveFormat=Timeseries  SampleTime=-1
  To Workspace22 : ToWorkspace  VariableName=Q_44  SaveFormat=Timeseries  SampleTime=-1
  To Workspace23 : ToWorkspace  VariableName=Q_34  SaveFormat=Timeseries  SampleTime=-1
  To Workspace24 : ToWorkspace  VariableName=Q_24  SaveFormat=Timeseries  SampleTime=-1
  To Workspace25 : ToWorkspace  VariableName=Q_14  SaveFormat=Timeseries  SampleTime=-1
  To Workspace26 : ToWorkspace  VariableName=Done_Out  SaveFormat=Timeseries  SampleTime=-1
  To Workspace27 : ToWorkspace  VariableName=C_1  SaveFormat=Timeseries  SampleTime=-1
  To Workspace28 : ToWorkspace  VariableName=C_  SaveFormat=Timeseries  SampleTime=-1
  To Workspace29 : ToWorkspace  VariableName=C_2  SaveFormat=Timeseries  SampleTime=-1
  To Workspace3 : ToWorkspace  VariableName=R_13  SaveFormat=Timeseries  SampleTime=-1
  To Workspace30 : ToWorkspace  VariableName=C_3  SaveFormat=Timeseries  SampleTime=-1
  To Workspace4 : ToWorkspace  VariableName=R_23  SaveFormat=Timeseries  SampleTime=-1
  To Workspace5 : ToWorkspace  VariableName=R_33  SaveFormat=Timeseries  SampleTime=-1
  To Workspace6 : ToWorkspace  VariableName=R_34  SaveFormat=Timeseries  SampleTime=-1
  To Workspace7 : ToWorkspace  VariableName=R_44  SaveFormat=Timeseries  SampleTime=-1
  To Workspace8 : ToWorkspace  VariableName=R_24  SaveFormat=Timeseries  SampleTime=-1
  To Workspace9 : ToWorkspace  VariableName=R_14  SaveFormat=Timeseries  SampleTime=-1
  ap_rst : hdlBasic/Gateway In  gui_display_data_type=Boolean  arith_type=Boolean  n_bits=16  bin_pt=14  preci_type=Single  exp_width=8  frac_width=24  rows=1  columns=1  quantization="Round  (unbiased: +/- Inf)"  overflow=Saturate  period=1  UseAsADC=off  ADCChannel='1'  interface=AXI4-Lite  automatic_assignment=on  address_offset=hex2dec('00')  intf_name='control'  intf_description=''  default_value=0  timing_constraint=None  locs_specified=off  LOCs={}  io_standard={}  inherit_from_input=off  hdl_port=on  XmcBlockStatus=1  maskContainerNames=group4  block_type=gatewayin  block_config=sysgen:gateway_in_config  block_width_w=590  block_height_w=620  block_width=640  block_height=850
  in_{5..8,11..13,21..23,31..33,41..43} (16 alike) : hdlBasic/Gateway In  gui_display_data_type=Fixed-point  arith_type=Signed (2's comp)  n_bits=16  bin_pt=12  preci_type=Single  exp_width=8  frac_width=24  rows=1  columns=1  quantization="Round  (unbiased: +/- Inf)"  overflow=Saturate  period=1  UseAsADC=off  ADCChannel='1'  interface=AXI4-Lite  automatic_assignment=on  address_offset=hex2dec('00')  intf_name='array_input'  intf_description=''  default_value=0  timing_constraint=None  locs_specified=off  LOCs={}  io_standard={}  inherit_from_input=off  hdl_port=on  XmcBlockStatus=1  maskContainerNames=group4  block_type=gatewayin  block_config=sysgen:gateway_in_config  block_width_w=590  block_height_w=620  block_width=640  block_height=850
  start_new : hdlBasic/Gateway In  gui_display_data_type=Boolean  arith_type=Boolean  n_bits=16  bin_pt=14  preci_type=Single  exp_width=8  frac_width=24  rows=1  columns=1  quantization="Round  (unbiased: +/- Inf)"  overflow=Saturate  period=1  UseAsADC=off  ADCChannel='1'  interface=AXI4-Lite  automatic_assignment=on  address_offset=hex2dec('00')  intf_name='control'  intf_description=''  default_value=0  timing_constraint=None  locs_specified=off  LOCs={}  io_standard={}  inherit_from_input=off  hdl_port=on  XmcBlockStatus=1  maskContainerNames=group4  block_type=gatewayin  block_config=sysgen:gateway_in_config  block_width_w=590  block_height_w=620  block_width=640  block_height=850
  wires:
  From Workspace/1 -> ap_rst/1  "ap_rst"
  Subsystem1/1 -> Subsystem Reference2/4  "sine_in"
  Subsystem Reference2/2 -> Subsystem Reference/3
  Delay2/1 -> Delay3/1, Subsystem Reference5/3  "angle"
  Subsystem2/1 -> Subsystem Reference5/4  "sine_in"
  Subsystem Reference2/1 -> Subsystem2/5, Subsystem Reference5/2, Subsystem Reference/2  "ap_start"
  Subsystem3/1 -> Subsystem Reference6/4  "sine_in"
  Subsystem Reference5/1 -> Subsystem3/5, Subsystem Reference6/2  "ap_start"
  Subsystem Reference/1 -> Subsystem Reference7/2  "ap_start"
  Subsystem Reference/2 -> Delay5/1, Subsystem Reference7/3  "angle"
  Delay5/1 -> Delay13/1, Subsystem Reference8/3  "angle"
  Subsystem Reference7/1 -> Subsystem Reference8/2, Subsystem Reference3/2  "ap_start"
  Subsystem Reference3/1 -> Subsystem Reference4/2  "ap_start"
  Delay6/1 -> Subsystem Reference13/3, Delay7/1  "angle"
  Delay3/1 -> Delay6/1, Subsystem Reference6/3  "angle"
  Subsystem Reference6/1 -> Subsystem4/5, Subsystem Reference13/2
  Delay7/1 -> Subsystem Reference14/3, Delay8/1  "angle"
  Delay8/1 -> Subsystem Reference15/3, Delay9/1  "angle"
  Subsystem Reference13/1 -> Subsystem Reference14/2, Subsystem6/5  "ap_start"
  Delay12/1 -> Subsystem Reference20/3  "angle"
  Delay11/1 -> Delay12/1, Subsystem Reference19/3  "angle"
  Delay10/1 -> Delay11/1, Subsystem Reference18/3  "angle"
  Delay13/1 -> Delay10/1, Subsystem Reference17/3  "angle"
  Subsystem Reference8/2 -> Subsystem Reference4/4
  Subsystem Reference7/2 -> Subsystem Reference3/3
  Subsystem Reference6/2 -> Subsystem Reference8/4
  Subsystem Reference5/2 -> Subsystem Reference7/4
  Subsystem Reference18/2 -> Subsystem Reference10/4
  Delay21/1 -> Subsystem Reference9/3, Delay18/1  "angle"
  Delay19/1 -> Delay20/1, Subsystem Reference11/3  "angle"
  Subsystem Reference19/2 -> Subsystem Reference11/4
  Subsystem Reference20/2 -> Subsystem Reference12/4
  Subsystem Reference10/1 -> Subsystem Reference11/2  "ap_start"
  Subsystem Reference9/1 -> Subsystem Reference10/2  "ap_start"
  Delay20/1 -> Subsystem Reference12/3  "angle"
  Delay18/1 -> Delay19/1, Subsystem Reference10/3  "angle"
  Subsystem Reference3/2 -> Delay21/1, Subsystem Reference4/3  "reset"
  Subsystem Reference4/1 -> Subsystem Reference9/2
  Subsystem Reference11/1 -> Subsystem Reference12/2  "ap_start"
  Subsystem Reference17/2 -> Subsystem Reference9/4
  ap_rst/1 -> Subsystem Reference/1, Subsystem Reference3/1, Subsystem Reference4/1, Subsystem Reference9/1, Subsystem Reference12/1, Subsystem Reference11/1, Subsystem Reference10/1, Subsystem Reference20/1, Subsystem Reference19/1, Subsystem Reference18/1, Subsystem Reference17/1, Subsystem Reference8/1, Subsystem Reference7/1, Subsystem Reference1/1, Subsystem Reference2/1, Subsystem Reference16/1, Subsystem Reference15/1, Subsystem Reference14/1, Subsystem Reference13/1, Subsystem Reference6/1, Subsystem Reference5/1  "reset"
  Subsystem Reference4/2 -> Register3/1
  Subsystem Reference4/4 -> Register3/2, Register9/2
  Register/1 -> R_11/1
  Subsystem Reference1/1 -> Subsystem Reference2/2, Subsystem1/5, Subsystem/5  "ap_start"
  Subsystem Reference1/2 -> Subsystem Reference2/3, Delay2/1  "angle"
  Register1/1 -> R_22/1
  Subsystem Reference/4 -> Register1/2
  Subsystem Reference/3 -> Register1/1
  Subsystem Reference3/4 -> Register2/2
  Register2/1 -> R_33/1
  Subsystem Reference3/3 -> Register2/1
  Register3/1 -> R_44/1
  Subsystem Reference9/2 -> Delay/1
  Subsystem Reference9/4 -> Subsystem11/2, Delay1/1
  Subsystem Reference10/4 -> Subsystem15/2, Delay14/1
  Subsystem Reference10/2 -> Delay4/1
  Subsystem Reference11/2 -> Register6/1
  Subsystem Reference11/4 -> Register6/2, Register16/2
  Register6/1 -> Q_43/1
  Subsystem Reference12/2 -> Register7/1
  Subsystem Reference12/4 -> Register17/2, Logical3/1, Register27/1, Register7/2
  Register7/1 -> Q_44/1
  Register8/1 -> R_12/1
  Subsystem Reference2/4 -> Register8/2
  Subsystem Reference2/3 -> Register8/1
  Register9/1 -> R_34/1
  Subsystem Reference4/3 -> Register9/1
  Register10/1 -> R_13/1
  Subsystem Reference5/3 -> Register10/1
  Subsystem Reference5/4 -> Register10/2
  Register11/1 -> R_14/1
  Subsystem Reference6/3 -> Register11/1
  Subsystem Reference6/4 -> Register11/2
  Register12/1 -> R_23/1
  Subsystem Reference7/3 -> Register12/1
  Subsystem Reference7/4 -> Register12/2
  Register13/1 -> R_24/1
  Subsystem Reference8/3 -> Register13/1
  Subsystem Reference8/4 -> Register13/2
  Subsystem Reference10/3 -> Q_32/1, Subsystem15/1
  Subsystem Reference11/3 -> Register16/1
  Register16/1 -> Q_33/1
  Subsystem Reference12/3 -> Register17/1
  Register17/1 -> Q_34/1
  Subsystem Reference13/4 -> Subsystem10/2
  Subsystem Reference13/3 -> Subsystem10/1, Q_11/1
  Subsystem Reference14/4 -> Subsystem17/2
  Subsystem Reference14/3 -> Q_12/1, Subsystem17/1
  Subsystem Reference15/3 -> Register20/1
  Subsystem Reference15/4 -> Register20/2
  Register20/1 -> Q_13/1
  Subsystem Reference16/3 -> Register21/1
  Subsystem Reference16/4 -> Register21/2
  Register21/1 -> Q_14/1
  Subsystem Reference17/4 -> Subsystem9/2
  Subsystem Reference17/3 -> Q_21/1, Subsystem9/1
  Subsystem Reference18/4 -> Subsystem16/2
  Subsystem Reference18/3 -> Q_22/1, Subsystem16/1
  Subsystem Reference19/3 -> Register24/1
  Subsystem Reference19/4 -> Register24/2
  Register24/1 -> Q_23/1
  Subsystem Reference20/3 -> Register25/1
  Subsystem Reference20/4 -> Register25/2
  Register25/1 -> Q_24/1
  Subsystem Reference13/2 -> Subsystem Reference17/4
  Subsystem Reference14/2 -> Subsystem Reference18/4
  Subsystem Reference15/2 -> Subsystem Reference19/4
  Subsystem Reference16/2 -> Subsystem Reference20/4
  Subsystem Reference19/1 -> Subsystem Reference20/2  "ap_start"
  Subsystem Reference18/1 -> Subsystem Reference19/2  "ap_start"
  Subsystem Reference17/1 -> Subsystem Reference18/2  "ap_start"
  Subsystem Reference8/1 -> Subsystem Reference17/2  "ap_start"
  R_13/1 -> To Workspace3/1, Display/1  "row_1_data"
  R_23/1 -> To Workspace4/1, Display1/1  "row_1_data"
  R_33/1 -> To Workspace5/1, Display2/1  "row_1_data"
  R_14/1 -> To Workspace9/1, Display3/1  "row_1_data"
  R_24/1 -> To Workspace8/1, Display4/1  "row_1_data"
  R_34/1 -> To Workspace6/1, Display5/1  "row_1_data"
  R_44/1 -> Display6/1, To Workspace7/1  "row_1_data"
  Q_31/1 -> Display7/1, To Workspace12/1  "row_1_data"
  Q_41/1 -> To Workspace13/1, Display8/1  "row_1_data"
  Q_21/1 -> To Workspace11/1, Display9/1  "row_1_data"
  Q_11/1 -> Display10/1, To Workspace10/1  "row_1_data"
  Q_12/1 -> To Workspace17/1, Display11/1  "row_1_data"
  Q_22/1 -> To Workspace16/1, Display12/1  "row_1_data"
  Q_32/1 -> To Workspace15/1, Display13/1  "row_1_data"
  Q_42/1 -> To Workspace14/1, Display14/1  "row_1_data"
  Q_43/1 -> To Workspace21/1, Display15/1  "row_1_data"
  Q_33/1 -> To Workspace20/1, Display16/1  "row_1_data"
  Q_23/1 -> To Workspace19/1, Display17/1  "row_1_data"
  Q_13/1 -> To Workspace18/1, Display18/1  "row_1_data"
  Q_44/1 -> To Workspace22/1, Display19/1  "row_1_data"
  Q_34/1 -> To Workspace23/1, Display20/1  "row_1_data"
  Q_24/1 -> To Workspace24/1, Display21/1  "row_1_data"
  Q_14/1 -> To Workspace25/1, Display22/1  "row_1_data"
  R_22/1 -> To Workspace2/1, Display23/1  "row_1_data"
  R_12/1 -> To Workspace1/1, Display24/1  "row_1_data"
  R_11/1 -> To Workspace/1, Display25/1  "row_1_data"
  Delay9/1 -> Subsystem Reference16/3  "angle"
  From Workspace6/1 -> in_11/1  "sine_in"
  From Workspace8/1 -> in_21/1  "sine_in"
  From Workspace9/1 -> in_31/1  "sine_in"
  From Workspace10/1 -> in_41/1  "sine_in"
  in_11/1 -> Subsystem/1
  in_21/1 -> Subsystem/2
  in_31/1 -> Subsystem/3
  in_41/1 -> Subsystem/4
  Subsystem/1 -> Subsystem Reference1/3
  in_32/1 -> Subsystem1/3
  in_22/1 -> Subsystem1/2
  in_42/1 -> Subsystem1/4
  in_12/1 -> Subsystem1/1
  From Workspace7/1 -> in_12/1  "sine_in"
  From Workspace12/1 -> in_32/1  "sine_in"
  From Workspace3/1 -> in_42/1  "sine_in"
  From Workspace11/1 -> in_22/1  "sine_in"
  in_33/1 -> Subsystem2/3
  in_23/1 -> Subsystem2/2
  in_43/1 -> Subsystem2/4
  in_13/1 -> Subsystem2/1
  From Workspace4/1 -> in_13/1  "sine_in"
  From Workspace13/1 -> in_33/1  "sine_in"
  From Workspace2/1 -> in_43/1  "sine_in"
  From Workspace5/1 -> in_23/1  "sine_in"
  in_7/1 -> Subsystem3/3
  in_6/1 -> Subsystem3/2
  in_8/1 -> Subsystem3/4
  in_5/1 -> Subsystem3/1
  From Workspace15/1 -> in_5/1  "sine_in"
  From Workspace17/1 -> in_7/1  "sine_in"
  From Workspace14/1 -> in_8/1  "sine_in"
  From Workspace16/1 -> in_6/1  "sine_in"
  Subsystem/2 -> Register26/1  "ap_start"
  Subsystem Reference1/4 -> Register/2
  Subsystem Reference1/3 -> Register/1  "ap_start"
  Register26/1 -> Subsystem Reference1/2
  Constant/1 -> Subsystem4/1
  Constant1/1 -> Subsystem4/2
  Constant3/1 -> Subsystem4/4
  Constant2/1 -> Subsystem4/3
  Subsystem4/1 -> Subsystem Reference13/4  "sine_in"
  Constant7/1 -> Subsystem6/4
  Constant5/1 -> Subsystem6/2
  Constant6/1 -> Subsystem6/3
  Constant4/1 -> Subsystem6/1
  Subsystem6/1 -> Subsystem Reference14/4  "sine_in"
  Constant8/1 -> Subsystem5/1
  Constant9/1 -> Subsystem5/2
  Subsystem Reference14/1 -> Subsystem Reference15/2, Subsystem5/5  "ap_start"
  Constant11/1 -> Subsystem5/4
  Constant10/1 -> Subsystem5/3
  Subsystem5/1 -> Subsystem Reference15/4  "sine_in"
  Constant12/1 -> Subsystem7/1
  Constant13/1 -> Subsystem7/2
  Subsystem Reference15/1 -> Subsystem7/5, Subsystem Reference16/2  "ap_start"
  Constant15/1 -> Subsystem7/4
  Constant14/1 -> Subsystem7/3
  Subsystem7/1 -> Subsystem Reference16/4  "sine_in"
  From Workspace1/1 -> start_new/1  "ap_rst"
  start_new/1 -> Logical3/2, Subsystem7/6, Subsystem5/6, Subsystem6/6, Subsystem4/6, Subsystem3/6, Subsystem2/6, Subsystem1/6, Subsystem/6  "reset"
  Register27/1 -> Q_1/1
  Logical3/1 -> Register27/2
  Q_1/1 -> To Workspace26/1, Display26/1  "row_1_data"
  Register28/1 -> MultAdd/3
  MultAdd/1 -> C_1/1, Register28/1
  Subsystem8/2 -> Register28/2
  Subsystem8/1 -> MultAdd/1
  From Workspace18/1 -> B_1/1  "sine_in"
  Delay/1 -> Q_41/1, Subsystem8/1
  Delay1/1 -> Subsystem8/2
  C_1/1 -> To Workspace27/1, Display27/1  "row_1_data"
  Subsystem10/2 -> Subsystem9/4
  Subsystem10/1 -> Subsystem9/3
  Subsystem Reference9/3 -> Q_31/1, Subsystem11/1
  Subsystem9/2 -> Subsystem11/4
  Subsystem9/1 -> Subsystem11/3
  Subsystem11/2 -> Subsystem8/4
  Subsystem11/1 -> Subsystem8/3
  Constant16/1 -> Subsystem10/4
  Constant17/1 -> Subsystem10/3
  Subsystem12/1 -> MultAdd1/1
  MultAdd1/1 -> C_2/1, Register4/1
  C_2/1 -> To Workspace28/1, Display28/1  "row_1_data"
  Register4/1 -> MultAdd1/3
  Subsystem12/2 -> Register4/2
  Subsystem13/1 -> MultAdd2/1
  MultAdd2/1 -> C_3/1, Register14/1
  C_3/1 -> To Workspace29/1, Display29/1  "row_1_data"
  Register14/1 -> MultAdd2/3
  Subsystem13/2 -> Register14/2
  Subsystem14/1 -> MultAdd3/1
  MultAdd3/1 -> C_4/1, Register18/1
  C_4/1 -> To Workspace30/1, Display30/1  "row_1_data"
  Register18/1 -> MultAdd3/3
  Subsystem14/2 -> Register18/2
  Delay4/1 -> Q_42/1, Subsystem12/1
  Delay14/1 -> Subsystem12/2
  Subsystem15/2 -> Subsystem12/4
  Subsystem15/1 -> Subsystem12/3
  Subsystem16/2 -> Subsystem15/4
  Subsystem16/1 -> Subsystem15/3
  Subsystem17/2 -> Subsystem16/4
  Subsystem17/1 -> Subsystem16/3
  Constant18/1 -> Subsystem17/4
  Constant19/1 -> Subsystem17/3
